simulink model "FOC_simu"  (R2018b)
settings: Solver=FixedStepDiscrete  StartTime=0.0  StopTime=inf  FixedStep=4e-6  RelTol=1e-3
undefined symbols (not defined in the file or in its folder): sigbuilder_block
libraries: simulink x7, powerlib x4
settings Model: Creator=Administrator  LastModifiedBy=nie.fei
settings DataIOCC: LimitDataPoints=on
settings OptimizationCC: BlockReduction=off  DefaultParameterBehavior=Inlined  DefaultUnderspecifiedDataType=single  LifeSpan=1
settings DebuggingCC: SignalInfNanChecking=warning  UnderspecifiedInitializationDetection=Classic  MergeDetectMultiDrivingBlocksExec=none  MultiTaskCondExecSysMsg=warning  MultiTaskRateTransMsg=warning  ParameterPrecisionLossMsg=none  SFUnexpectedBacktrackingDiag=warning  SFNoUnconditionalDefaultTransitionDiag=warning  SFExecutionAtInitializationDiag=none
settings HardwareCC: ProdBitPerPointer=32  ProdBitPerSizeT=32  ProdBitPerPtrDiffT=32  ProdLargestAtomicInteger=Long  ProdLargestAtomicFloat=Double  ProdWordSize=32  ProdHWDeviceType=ARM Compatible->ARM Cortex
settings ModelReferenceCC: PropagateSignalLabelsOutOfModel=off
settings SFSimCC: SimUseLocalCustomCode=off  MATLABDynamicMemAlloc=off
settings RTWCC: SystemTargetFile=ert.tlc  GenCodeOnly=on  PackageName=AccPedal  TemplateMakefile=ert_default_tmf  GenerateReport=on  RTWVerbose=off  RTWUseLocalCustomCode=off  IncludeHyperlinkInReport=on  LaunchReport=on
settings CodeAppCC: IgnoreCustomStorageClasses=off  MaxIdLength=63  StateflowObjectComments=on
settings ERTTargetCC: TargetLangStandard=C99 (ISO)  MultiwordLength=2048  SupportNonFinite=off  ExtModeTransport=1  ExtModeMexFile=ext_serial_win32_comm  ERTCustomFileTemplate=example_file_process.tlc  ConvertIfToSwitch=off  SuppressUnreachableDefaultCases=off
settings ConfigComp: CovMetricSettings=dw  CovHtmlReporting=on  CovSaveCumulativeToWorkspaceVar=on  CovSaveSingleToWorkspaceVar=on  CovExternalEMLEnable=off  DVMaxProcessTime=600  DVMaxTestCaseSteps=500  DVTestSuiteOptimization=CombinedObjectives (Nonlinear Extended)  DVSaveReport=on
settings SimscapeCC: SimscapeNormalizeSystem=off

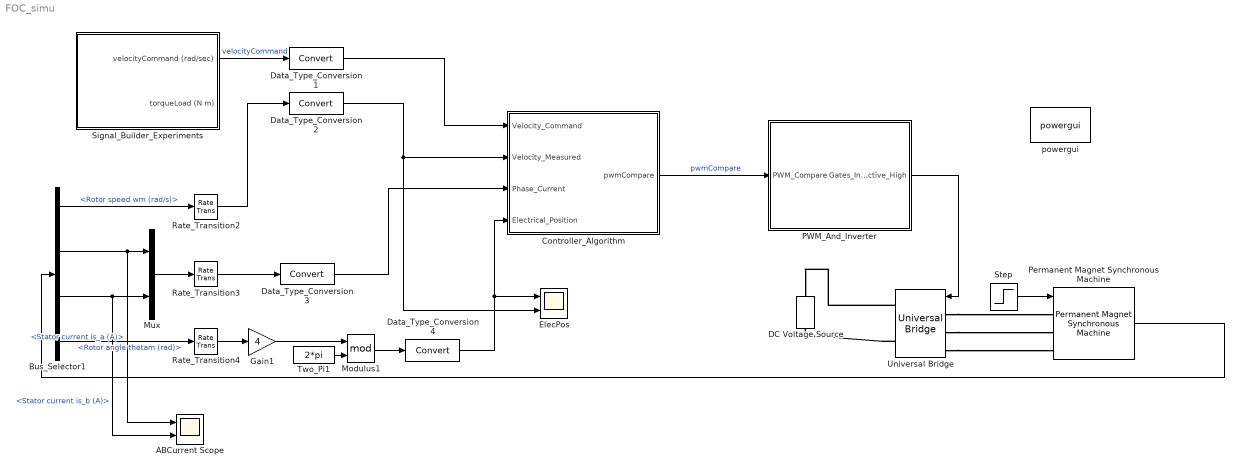
== system FOC_simu ==
  ABCurrent Scope : Scope  NumInputPorts=2
  Bus_Selector1 : BusSelector  OutputSignals=Rotor speed wm (rad/s),Stator current is_a (A),Stator current is_b (A),Rotor angle thetam (rad)
  Controller_Algorithm : Subsystem
  DC Voltage Source : powerlib/Electrical Sources/DC Voltage Source  Amplitude=24  Measurements=None
      settings: AttributesFormatString=%<Amplitude>
  Data_Type_Conversion{1..4} (4 alike) : DataTypeConversion
  ElecPos : Scope  NumInputPorts=2
  Gain1 : Gain  Gain=4
  Modulus1 : Math  Operator=mod  SaturateOnIntegerOverflow=on
  Mux : Mux  Inputs=2
  PWM_And_Inverter : Subsystem  VariantControl=variantPwm == enumPwm.behavior
      mask Display:
      | image('pwmAndInverterMask.png')
      | port_label('input',1,'En')
      | port_label('input',2,'Compare')
      | text(0.98, 0.88, 'G', 'HorizontalAlignment', 'Right')
      | text(0.98, 0.62, 'A', 'HorizontalAlignment', 'Right')
      | text(0.98, 0.38, 'B', 'HorizontalAlignment', 'Right')
      | text(0.98, 0.12, 'C', 'HorizontalAlignment', 'Right')
  Permanent Magnet Synchronous Machine : powerlib/Machines/Permanent Magnet Synchronous Machine  NbPhases=3  FluxDistribution=Sinusoidal  RotorType=Salient-pole  MechanicalLoad=Torque Tm  PresetModel=No  ShowDetailedParameters=on  MeasurementBus=off  Resistance=0.9  Inductance=8.5e-3  dqInductances=[0.0011 0.0011]  La=0.000395  MachineConstant=Flux linkage established by magnets (V.s)  Flux=0.0057  VoltageCst=4.1355  TorqueCst=0.0342  Flat=120  Mechanical=[2.400927680000000e-06 1.333630000000000e-05 4 0]  PolePairs=4  InitialConditions=[0,0, 0,0]  InitialConditions5ph=[0 0 0 0 0 0]  TsPowergui=0  TsBlock=-1  RefAngle=Aligned with phase A axis (original Park)
      settings: SourceProductName=Simscape Power Systems
  Rate_Transition2 : RateTransition  Integrity=off  Deterministic=off
  Rate_Transition3 : RateTransition  Integrity=off  Deterministic=off
  Rate_Transition4 : RateTransition  Integrity=off  Deterministic=off
  Signal_Builder_Experiments : Subsystem  Tag=STV Subsys  LoadFcn=sigbuilder_block('load');  StartFcn=sigbuilder_block('start');  StopFcn=sigbuilder_block('stop');  ClipboardFcn=sigbuilder_block('clipboard');  mask(Sigbuilder block){tuvar=[0:10]}
      mask init:
      | if ~strcmp(get_param(bdroot(gcb),'SimulationStatus'),'stopped'),tuvar = sigbuilder_block('maskInit'); end
      settings: CopyFcn=sigbuilder_block('copy');  DeleteFcn=sigbuilder_block('delete');  ModelCloseFcn=sigbuilder_block('modelClose');  PreSaveFcn=sigbuilder_block('preSave');  PauseFcn=sigbuilder_block('pause');  ContinueFcn=sigbuilder_block('continue');  NameChangeFcn=sigbuilder_block('namechange');  OpenFcn=sigbuilder_block('open',[0 30 1024.5 487.5 ]);  CloseFcn=sigbuilder_block('close');
      mask Display: plot(0, 0, 100, 100,[2, 2, 32, 32, 2], [68, 8, 8, 68, 68],[32, 2], [38, 38], [32, 19, 2],[53, 60, 44], [32, 17, 17, 2],[16, 16, 31, 31]);txt = getActiveGroup(gcbh);text(2, 100, txt,'verticalAlignment', 'top');
  Step : Step  Time=0.01  After=0
  Two_Pi1 : Constant  Value=2*pi  OutDataTypeStr=Inherit: Inherit via back propagation
  Universal Bridge : powerlib/Power Electronics/Universal Bridge  Arms=3  SnubberResistance=1e5  SnubberCapacitance=inf  Device=IGBT / Diodes  Ron=1e-3  Lon=0  ForwardVoltages="[  0  0  ]"  ForwardVoltage=0  GTOparameters=[ 10e-6 , 20e-6 ]  IGBTparameters=[ 1e-6 , 2e-6 ]  Measurements=None  Measurements_2=None  converterType=Rectifier
  powergui : powerlib/powergui  Priority=1  SimulationMode=Discrete  SampleTime=4.0e-6  frequency=60  Iterations=50  frequencyindice=0  Pbase=100e6  ErrMax=1e-4  UnitsV=kV  UnitsW=MW  buscounter=0  FunctionMessages=off  echomessages=off  EnableUseOfTLC=off  CurrentSourceSwitches=off  DisableSnubberDevices=off  DisableRonSwitches=off  DisableVfSwitches=off  DisplayEquations=off  SolverType=Tustin/Backward Euler (TBE)  Interpol=off  ExternalGateDelay=off  methode=off  Ts=0  x0status=blocks  SPID=off  SwTol=0  HookPort=off  RestoreLinks=warning  ResistiveCurrentMeasurement=off  Frange=[0:2:500]  Ylog=off  Xlog=on  ShowGrid=off  save=off  variable=ZData  structure=0  ZoomFFT=on  StartTime=0.0  cycles=1  DisplayStyle=1  fundamental=60  FreqAxis=off  MaxFrequency=1000  frequencyindicesteady=1  RmsSteady=1  display=off
  wires:
  Step/1 -> Permanent Magnet Synchronous Machine/1
  Permanent Magnet Synchronous Machine/1 -> Bus_Selector1/1
  Rate_Transition4/1 -> Gain1/1
  Bus_Selector1/2 -> Mux/1, ABCurrent Scope/1  "<Stator current is_a (A)>"
  Mux/1 -> Rate_Transition3/1
  Bus_Selector1/3 -> Mux/2, ABCurrent Scope/2  "<Stator current is_b (A)>"
  Data_Type_Conversion3/1 -> Controller_Algorithm/3(Phase_Current)
  Rate_Transition3/1 -> Data_Type_Conversion3/1
  Bus_Selector1/4 -> Rate_Transition4/1  "<Rotor angle thetam (rad)>"
  Bus_Selector1/1 -> Rate_Transition2/1  "<Rotor speed wm (rad/s)>"
  Rate_Transition2/1 -> Data_Type_Conversion2/1
  Signal_Builder_Experiments/1(velocityCommand (rad/sec)) -> Data_Type_Conversion1/1  "velocityCommand"
  Gain1/1 -> Modulus1/1
  Modulus1/1 -> Data_Type_Conversion4/1
  Controller_Algorithm/1(pwmCompare) -> PWM_And_Inverter/1(PWM_Compare)  "pwmCompare"
  PWM_And_Inverter/1(Gates_Individual_Active_High) -> Universal Bridge/1
  Data_Type_Conversion1/1 -> Controller_Algorithm/1(Velocity_Command)
  Data_Type_Conversion4/1 -> ElecPos/1, Controller_Algorithm/4(Electrical_Position)
  Two_Pi1/1 -> Modulus1/2
  Data_Type_Conversion2/1 -> ElecPos/2, Controller_Algorithm/2(Velocity_Measured)
  connections:
  Universal Bridge/LConn1 -- Permanent Magnet Synchronous Machine/LConn1
  Universal Bridge/RConn1 -- DC Voltage Source/RConn1
  Universal Bridge/RConn2 -- DC Voltage Source/LConn1
  Universal Bridge/LConn2 -- Permanent Magnet Synchronous Machine/LConn2
  Universal Bridge/LConn3 -- Permanent Magnet Synchronous Machine/LConn3

== system FOC_simu/Controller_Algorithm ==
  Velocity_Command : Inport  OutDataTypeStr=single
  Velocity_Measured : Inport  Port=2  OutDataTypeStr=single
  Phase_Current : Inport  Port=3  OutDataTypeStr=single
  Electrical_Position : Inport  Port=4  OutDataTypeStr=single
  CurrentControl : Subsystem  TreatAsAtomicUnit=on  SystemSampleTime=200e-6  RTWFcnName=CurrentControl_Co  RTWFileName=CurrentControl
      settings: RTWSystemCode=Nonreusable function  RTWFcnNameOpts=User specified  RTWFileNameOpts=User specified
      settings: AttributesFormatString=|
      | ---------------------------------------
      | SampeTime = %<SystemSampleTime>
  SpeedControl : Subsystem  TreatAsAtomicUnit=on  SystemSampleTime=0.01  RTWFcnName=SpeedControl_Co  RTWFileName=SpeedControl
      settings: RTWSystemCode=Nonreusable function  RTWFcnNameOpts=User specified  RTWFileNameOpts=User specified
      settings: AttributesFormatString=|
      | ---------------------------------------
      | SampeTime = %<SystemSampleTime>
  pwmCompare : Outport
  wires:
  Velocity_Command/1 -> SpeedControl/1(Velocity_Command)
  Velocity_Measured/1 -> SpeedControl/2(Velocity_Measured)  "speed"
  Phase_Current/1 -> CurrentControl/1(Phase_Current)
  Electrical_Position/1 -> CurrentControl/3(Electrical_Position)
  CurrentControl/1(pwmCompare) -> pwmCompare/1
  SpeedControl/1(current_Iq) -> CurrentControl/2(current_Iq)

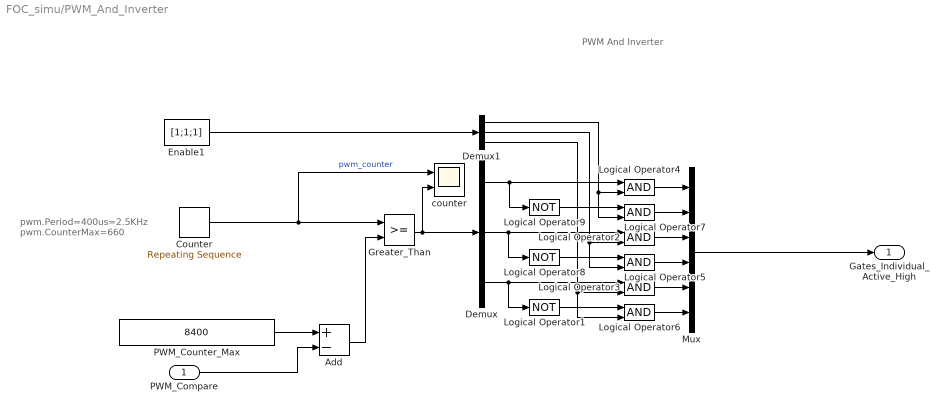
== system FOC_simu/PWM_And_Inverter ==
  note: pwm.Period=400us=2.5KHz
      | pwm.CounterMax=660
  note: PWM And Inverter
  PWM_Compare : Inport
  Add : Sum  Inputs=+-  OutDataTypeStr=Inherit: Same as first input
  Counter : simulink/Sources/Repeating Sequence  rep_seq_t=0.00005 * [0 0.5 1]  rep_seq_y=8400 * [0 1 0]
      settings: AttributesFormatString=|
      | ---------------------------------------
      | Time = %<rep_seq_t>
      | Values = %<rep_seq_y>
  Demux : Demux  Outputs=3
  Demux1 : Demux  Outputs=3
  Enable1 : Constant  Value=[1;1;1]
  Greater_Than : RelationalOperator  OutDataTypeStr=boolean  RndMeth=Nearest
  Logical Operator1 : Logic  Operator=NOT  IconShape=distinctive  AllPortsSameDT=off  OutDataTypeStr=boolean
  Logical Operator{2..7} (6 alike) : Logic  IconShape=distinctive  AllPortsSameDT=off  OutDataTypeStr=boolean
  Logical Operator8 : Logic  Operator=NOT  IconShape=distinctive  AllPortsSameDT=off  OutDataTypeStr=boolean
  Logical Operator9 : Logic  Operator=NOT  IconShape=distinctive  AllPortsSameDT=off  OutDataTypeStr=boolean
  Mux : Mux  Inputs=6
  PWM_Counter_Max : Constant  Value=8400  OutDataTypeStr=uint16
  counter : Scope  NumInputPorts=2
  Gates_Individual_Active_High : Outport
  wires:
  Mux/1 -> Gates_Individual_Active_High/1
  Counter/1 -> counter/1, Greater_Than/1  "pwm_counter"
  Demux/2 -> Logical Operator2/1, Logical Operator8/1
  Logical Operator1/1 -> Logical Operator6/1
  Logical Operator3/1 -> Mux/5
  Demux/1 -> Logical Operator9/1, Logical Operator4/1
  Logical Operator5/1 -> Mux/4
  Logical Operator6/1 -> Mux/6
  Demux1/1 -> Logical Operator4/2, Logical Operator7/2
  Demux1/3 -> Logical Operator6/2, Logical Operator3/2
  Logical Operator9/1 -> Logical Operator7/1
  Demux1/2 -> Logical Operator5/2, Logical Operator2/2
  Logical Operator8/1 -> Logical Operator5/1
  Logical Operator7/1 -> Mux/2
  Logical Operator4/1 -> Mux/1
  Demux/3 -> Logical Operator3/1, Logical Operator1/1
  Logical Operator2/1 -> Mux/3
  Enable1/1 -> Demux1/1
  Greater_Than/1 -> counter/2, Demux/1
  PWM_Compare/1 -> Add/2
  PWM_Counter_Max/1 -> Add/1
  Add/1 -> Greater_Than/2

== system FOC_simu/Signal_Builder_Experiments ==
  Demux : Demux  Tag=STV Demux  Outputs=2
  FromWs : FromWorkspace  Tag=STV FromWs  VariableName=tuvar
      SigBuilderData=|
      | dataSet(1).timeRange = [0 4.5]
      | dataSet(1).name = '150 rad/sec, no load'
      | dataSet(2).timeRange = [0 1]
      | dataSet(2).name = '+/-1 150 rad/sec, no load'
      | sbobj.Name = 'Signal Builder'
      | sbobj.Groups(1).Name = '150 rad/sec, no load'
      | sbobj.Groups(1).Signals(1).Name = 'velocityCommand (rad/sec)'
      | sbobj.Groups(1).Signals(1).XData = [0 0.05 0.5 0.7 1.1 3.7 3.9 3.9 4.3 4.3 4.5]
      | sbobj.Groups(1).Signals(1).YData = [0 0 150 200 200 200 200 100 100 150 150]
      | sbobj.Groups(1).Signals(2).Name = 'torqueLoad (N m)'
      | sbobj.Groups(1).Signals(2).XData = [0 4.5]
      | sbobj.Groups(1).Signals(2).YData = [0 0]
      | sbobj.Groups(1).TimeRange = [0 4.5]
      | sbobj.Groups(2).Name = '+/-1 150 rad/sec, no load'
      | sbobj.Groups(2).Signals(1).Name = 'velocityCommand (rad/sec)'
      | sbobj.Groups(2).Signals(1).XData = [0 0.05 0.05 0.5 0.5 0.8 0.8 1]
      | sbobj.Groups(2).Signals(1).YData = [0 0 150 150 -150 -150 0 0]
      | sbobj.Groups(2).Signals(2).Name = 'torqueLoad (N m)'
      | sbobj.Groups(2).Signals(2).XData = [0 1]
      | sbobj.Groups(2).Signals(2).YData = [0 0]
      | sbobj.Groups(2).TimeRange = [0 1]
  velocityCommand (rad/sec) : Outport  Tag=STV Outport
  torqueLoad (N m) : Outport  Tag=STV Outport  Port=2
  wires:
  Demux/2 -> torqueLoad (N m)/1
  Demux/1 -> velocityCommand (rad/sec)/1
  FromWs/1 -> Demux/1

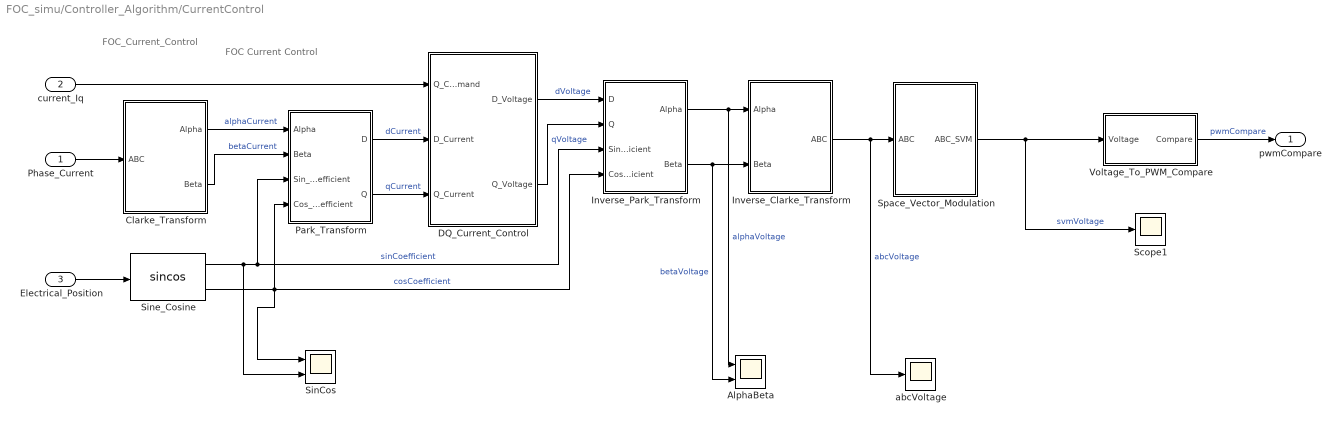
== system FOC_simu/Controller_Algorithm/CurrentControl ==
  note: FOC Current Control
  note: FOC_Current_Control
  Phase_Current : Inport  OutDataTypeStr=single
  current_Iq : Inport  Port=2
  Electrical_Position : Inport  Port=3  OutDataTypeStr=single
  AlphaBeta : Scope  NumInputPorts=2
  Clarke_Transform : Subsystem
      mask Display:
      | port_label('input',1,'ABC')
      | port_label('output',1,'\alpha','texmode', 'on')
      | port_label('output',2,'\beta','texmode', 'on')
  DQ_Current_Control : Subsystem
  Inverse_Clarke_Transform : Subsystem  VariantControl=INVERSE_CLARKE_TRANSFORM
      mask Display:
      | port_label('input',1,'\alpha','texmode', 'on')
      | port_label('input',2,'\beta','texmode', 'on')
      | port_label('output',1,'ABC')
  Inverse_Park_Transform : Subsystem
      mask Display:
      | port_label('input',1,'D')
      | port_label('input',2,'Q')
      | port_label('input',3,'Sin')
      | port_label('input',4,'Cos')
      | port_label('output',1,'\alpha','texmode', 'on')
      | port_label('output',2,'\beta','texmode', 'on')
  Park_Transform : Subsystem
      mask Display:
      | port_label('input',1,'\alpha','texmode', 'on')
      | port_label('input',2,'\beta','texmode', 'on')
      | port_label('input',3,'Sin')
      | port_label('input',4,'Cos')
      | port_label('output',1,'D')
      | port_label('output',2,'Q')
  Scope1 : Scope
  SinCos : Scope  NumInputPorts=2
  Sine_Cosine : Trigonometry  Operator=sincos
  Space_Vector_Modulation : Subsystem  VariantControl=SpaceVectorModulation_JB
      mask Display:
      | plot([0.000 0.020 0.041 0.061 0.082 0.102 0.122 0.143 0.163 0.184 0.204 0.224 0.245 0.265 0.286 0.306 0.327 0.347 0.367 0.388 0.408 0.429 0.449 0.469 0.490 0.510 0.531 0.551 0.571 0.592 0.612 0.633 0.653 0.673 0.694 0.714 0.735 0.755 0.776 0.796 0.816 0.837 0.857 0.878 0.898 0.918 0.939 0.959 0.980 1.000 ], ...
      |      [0.500 0.586 0.671 0.753 0.831 0.858 0.875 0.885 0.890 0.887 0.879 0.864 0.844 0.855 0.872 0.884 0.889 0.888 0.881 0.867 0.847 0.793 0.713 0.629 0.543 0.457 0.371 0.287 0.207 0.153 0.133 0.119 0.112 0.111 0.116 0.128 0.145 0.156 0.136 0.121 0.113 0.110 0.115 0.125 0.142 0.169 0.247 0.329 0.414 0.500 ])
  Voltage_To_PWM_Compare : Subsystem
  abcVoltage : Scope
  pwmCompare : Outport
  wires:
  Clarke_Transform/2(Beta) -> Park_Transform/2(Beta)  "betaCurrent"
  Inverse_Clarke_Transform/1(ABC) -> abcVoltage/1, Space_Vector_Modulation/1(ABC)  "abcVoltage"
  Phase_Current/1 -> Clarke_Transform/1(ABC)
  Electrical_Position/1 -> Sine_Cosine/1
  Inverse_Park_Transform/2(Beta) -> AlphaBeta/2, Inverse_Clarke_Transform/2(Beta)  "betaVoltage"
  Sine_Cosine/1 -> Park_Transform/3(Sin_Coefficient), Inverse_Park_Transform/3(Sin_Coefficient), SinCos/2  "sinCoefficient"
  Space_Vector_Modulation/1(ABC_SVM) -> Voltage_To_PWM_Compare/1(Voltage), Scope1/1  "svmVoltage"
  Park_Transform/1(D) -> DQ_Current_Control/2(D_Current)  "dCurrent"
  Sine_Cosine/2 -> SinCos/1, Park_Transform/4(Cos_Coefficient), Inverse_Park_Transform/4(Cos_Coefficient)  "cosCoefficient"
  Inverse_Park_Transform/1(Alpha) -> AlphaBeta/1, Inverse_Clarke_Transform/1(Alpha)  "alphaVoltage"
  Clarke_Transform/1(Alpha) -> Park_Transform/1(Alpha)  "alphaCurrent"
  Park_Transform/2(Q) -> DQ_Current_Control/3(Q_Current)  "qCurrent"
  Voltage_To_PWM_Compare/1(Compare) -> pwmCompare/1  "pwmCompare"
  DQ_Current_Control/1(D_Voltage) -> Inverse_Park_Transform/1(D)  "dVoltage"
  DQ_Current_Control/2(Q_Voltage) -> Inverse_Park_Transform/2(Q)  "qVoltage"
  current_Iq/1 -> DQ_Current_Control/1(Q_Command)

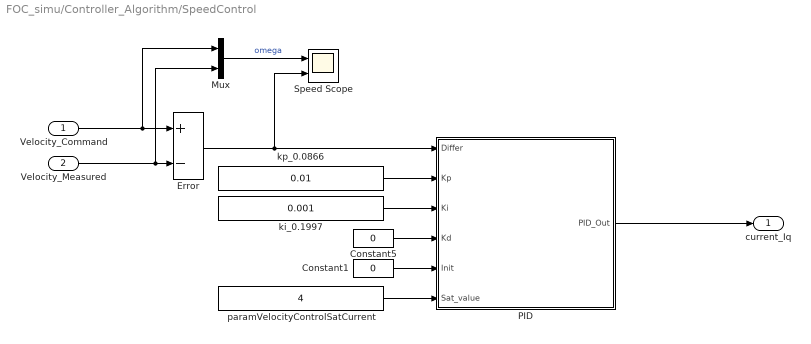
== system FOC_simu/Controller_Algorithm/SpeedControl ==
  Velocity_Command : Inport  OutDataTypeStr=single
  Velocity_Measured : Inport  Port=2  OutDataTypeStr=single
  Constant1 : Constant  Value=0  OutDataTypeStr=boolean  SampleTime=-1
  Constant5 : Constant  Value=0  OutDataTypeStr=Inherit: Inherit via back propagation  SampleTime=-1
  Error : Sum  Inputs=+-
  Mux : Mux  Inputs=2
  PID : Subsystem
  Speed Scope : Scope  NumInputPorts=2
  ki_0.1997 : Constant  Value=0.001  OutDataTypeStr=Inherit: Inherit via back propagation  SampleTime=-1
  kp_0.0866 : Constant  Value=0.01  OutDataTypeStr=Inherit: Inherit via back propagation  SampleTime=-1
  paramVelocityControlSatCurrent : Constant  Value=4  OutDataTypeStr=Inherit: Inherit via back propagation  SampleTime=-1
  current_Iq : Outport
  wires:
  PID/1(PID_Out) -> current_Iq/1
  ki_0.1997/1 -> PID/3(Ki)
  kp_0.0866/1 -> PID/2(Kp)
  Velocity_Measured/1 -> Mux/2, Error/2
  Error/1 -> Speed Scope/2, PID/1(Differ)
  Constant5/1 -> PID/4(Kd)
  Constant1/1 -> PID/5(Init)
  paramVelocityControlSatCurrent/1 -> PID/6(Sat_value)
  Mux/1 -> Speed Scope/1  "omega"
  Velocity_Command/1 -> Mux/1, Error/1

== system FOC_simu/Controller_Algorithm/CurrentControl/Clarke_Transform ==
  note: Clarke Transform
  note: Converts balanced three-phase quantities into balanced two-phase quantities.
      | The A and B phases are converted to the direct axis (alpha) component and the quadrature axis (beta) component.
      | The alpha and beta components are still dependent on time and speed.
  ABC : Inport
  A : Selector  IndexMode=Zero-based  InputPortWidth=2  IndexOptions=Index vector (dialog)  Indices=0  OutputSizes=1
  Add : Sum  OutDataTypeStr=Inherit: Same as first input
  Alpha_Gain : Gain  Gain=1/sqrt(3)
  B : Selector  IndexMode=Zero-based  InputPortWidth=2  IndexOptions=Index vector (dialog)  Indices=1  OutputSizes=1
  Beta_Gain : Gain  Gain=2/sqrt(3)
  Alpha : Outport
  Beta : Outport  Port=2
  wires:
  Add/1 -> Beta/1
  B/1 -> Beta_Gain/1
  Beta_Gain/1 -> Add/2
  ABC/1 -> A/1, B/1
  Alpha_Gain/1 -> Add/1
  A/1 -> Alpha_Gain/1, Alpha/1

== system FOC_simu/Controller_Algorithm/CurrentControl/DQ_Current_Control ==
  note: DQ Current Control
  Q_Command : Inport
  D_Current : Inport  Port=2
  Q_Current : Inport  Port=3
  Constant1 : Constant  Value=0.09  OutDataTypeStr=Inherit: Inherit via back propagation  SampleTime=-1
  Constant5 : Constant  Value=1.2  OutDataTypeStr=Inherit: Inherit via back propagation  SampleTime=-1
  D_Command : Constant  Value=0  OutDataTypeStr=single  SampleTime=-1
  D_Current_Control : Subsystem
  Q_Current_Control : Subsystem
  D_Voltage : Outport
  Q_Voltage : Outport  Port=2
  wires:
  Q_Current_Control/1(Voltage_Vq) -> Q_Voltage/1  "VQ"
  D_Current_Control/1(Voltage_Vd) -> D_Voltage/1  "VD"
  D_Command/1 -> D_Current_Control/1(Current_Command)  "IDcmd"
  Q_Command/1 -> Q_Current_Control/1(Current_Command)  "IQcmd"
  Q_Current/1 -> Q_Current_Control/2(Current_Measured)  "IQmea"
  D_Current/1 -> D_Current_Control/2(Current_Measured)  "IDmea"
  Constant5/1 -> Q_Current_Control/3(Current_Kp), D_Current_Control/3(Current_Kp)
  Constant1/1 -> Q_Current_Control/4(Current_Ki), D_Current_Control/4(Current_Ki)

== system FOC_simu/Controller_Algorithm/CurrentControl/Inverse_Clarke_Transform ==
  note: Inverse Clarke Transform
  note: Converts direct axis (alpha) component and the quadrature axis (beta) component to balanced three-phase quantities
      | The alpha and beta components are dependent on time and speed.
  Alpha : Inport
  Beta : Inport  Port=2
  Add : Sum  Inputs=-+  OutDataTypeStr=Inherit: Same as first input
  Add1 : Sum  Inputs=--  OutDataTypeStr=Inherit: Same as first input
  Gain : Gain  Gain=1/2
  Gain1 : Gain  Gain=sqrt(3)/2
  Mux : Mux  Inputs=3
  ABC : Outport
  wires:
  Gain/1 -> Add1/1, Add/1
  Gain1/1 -> Add1/2, Add/2
  Add/1 -> Mux/2
  Add1/1 -> Mux/3
  Beta/1 -> Gain1/1
  Alpha/1 -> Mux/1, Gain/1
  Mux/1 -> ABC/1

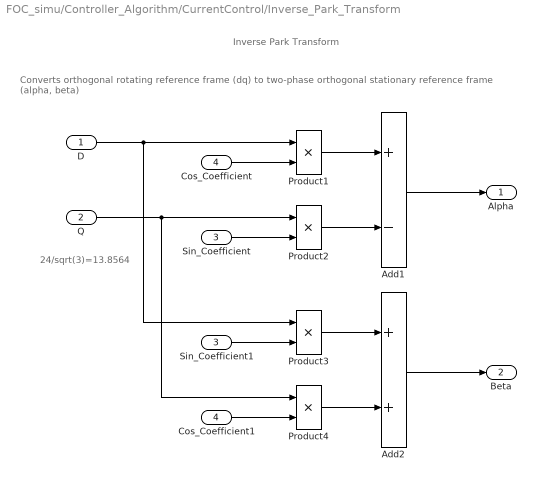
== system FOC_simu/Controller_Algorithm/CurrentControl/Inverse_Park_Transform ==
  note: Inverse Park Transform
  note: Converts orthogonal rotating reference frame (dq) to two-phase orthogonal stationary reference frame (alpha, beta)
  note: 24/sqrt(3)=13.8564
  D : Inport
  Q : Inport  Port=2
  Sin_Coefficient : Inport  Port=3
  Cos_Coefficient : Inport  Port=4
  Add1 : Sum  Inputs=+-  OutDataTypeStr=Inherit: Same as first input
  Add2 : Sum  OutDataTypeStr=Inherit: Same as first input
  Cos_Coefficient1 : InportShadow  Port=4
  Product{1..4} (4 alike) : Product  RndMeth=Simplest
  Sin_Coefficient1 : InportShadow  Port=3
  Alpha : Outport
  Beta : Outport  Port=2
  wires:
  Add2/1 -> Beta/1
  Add1/1 -> Alpha/1
  Product3/1 -> Add2/1
  Product4/1 -> Add2/2
  Product1/1 -> Add1/1
  Product2/1 -> Add1/2
  Cos_Coefficient1/1 -> Product4/2
  Sin_Coefficient/1 -> Product2/2
  D/1 -> Product3/1, Product1/1
  Q/1 -> Product2/1, Product4/1
  Sin_Coefficient1/1 -> Product3/2
  Cos_Coefficient/1 -> Product1/2

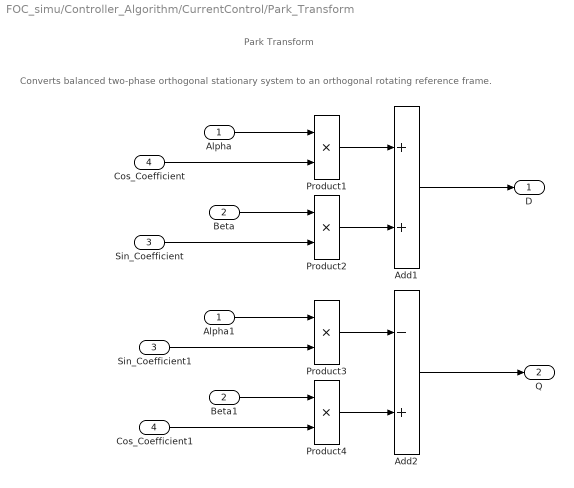
== system FOC_simu/Controller_Algorithm/CurrentControl/Park_Transform ==
  note: Park Transform
  note: Converts balanced two-phase orthogonal stationary system to an orthogonal rotating reference frame.
  Alpha : Inport
  Beta : Inport  Port=2
  Sin_Coefficient : Inport  Port=3
  Cos_Coefficient : Inport  Port=4
  Add1 : Sum  OutDataTypeStr=Inherit: Same as first input
  Add2 : Sum  Inputs=-+  OutDataTypeStr=Inherit: Same as first input
  Alpha1 : InportShadow
  Beta1 : InportShadow  Port=2
  Cos_Coefficient1 : InportShadow  Port=4
  Product{1..4} (4 alike) : Product  RndMeth=Simplest
  Sin_Coefficient1 : InportShadow  Port=3
  D : Outport
  Q : Outport  Port=2
  wires:
  Product3/1 -> Add2/1
  Product4/1 -> Add2/2
  Product1/1 -> Add1/1
  Product2/1 -> Add1/2
  Alpha1/1 -> Product3/1
  Sin_Coefficient1/1 -> Product3/2
  Cos_Coefficient1/1 -> Product4/2
  Beta1/1 -> Product4/1
  Alpha/1 -> Product1/1
  Cos_Coefficient/1 -> Product1/2
  Beta/1 -> Product2/1
  Sin_Coefficient/1 -> Product2/2
  Add1/1 -> D/1
  Add2/1 -> Q/1

== system FOC_simu/Controller_Algorithm/CurrentControl/Space_Vector_Modulation ==
  note: Space Vector Modulation
  ABC : Inport
  Add : Sum
  Add1 : Sum  Inputs=+-
  Gain : Gain  Gain=0.5  OutDataTypeStr=Inherit: Same as input
  Max : MinMax  Function=max
  Min : MinMax
  ABC_SVM : Outport
  wires:
  Add/1 -> Gain/1
  Max/1 -> Add/1
  Min/1 -> Add/2
  Gain/1 -> Add1/2
  ABC/1 -> Min/1, Max/1, Add1/1
  Add1/1 -> ABC_SVM/1

== system FOC_simu/Controller_Algorithm/CurrentControl/Voltage_To_PWM_Compare ==
  note: paramPwmCompareMax=660
  note: -12~+12
  note: ==>paramPwmComparePerVolt=27.5==>-330~+330
  note: 330
  note: 0~660
  note: Voltage To PWM Compare
  note: ==>paramPwmComparePerVolt=350==>-4200~+4200
  Voltage : Inport
  Add : Sum  OutDataTypeStr=Inherit: Inherit via back propagation
  Data_Type_Conversion : DataTypeConversion  OutDataTypeStr=uint16  LockScale=on
  Saturation : Saturate  UpperLimit=8400  LowerLimit=0
      settings: AttributesFormatString=|
      | --------------------------------
      | Upper Limit = %<UpperLimit>
      | Lower Limit = %<LowerLimit>
  Slope : Gain  Gain=350
      settings: AttributesFormatString=|
      | ----------------------------------------
      | Gain = %<Gain>
  paramPwmCompareAtZeroVolt : Constant  Value=4200  OutDataTypeStr=Inherit: Inherit via back propagation  SampleTime=-1
  Compare : Outport
  wires:
  Data_Type_Conversion/1 -> Compare/1  "pwmCompare"
  Voltage/1 -> Slope/1  "phaseVoltage"
  Slope/1 -> Add/1
  Saturation/1 -> Data_Type_Conversion/1
  paramPwmCompareAtZeroVolt/1 -> Add/2
  Add/1 -> Saturation/1

== system FOC_simu/Controller_Algorithm/SpeedControl/PID ==
  Differ : Inport  OutDataTypeStr=single
  Kp : Inport  Port=2  OutDataTypeStr=single
  Ki : Inport  Port=3  OutDataTypeStr=single
  Kd : Inport  Port=4  OutDataTypeStr=single
  Init : Inport  Port=5  OutDataTypeStr=boolean
  Sat_value : Inport  Port=6  OutDataTypeStr=single
  Delay6 : Delay  DelayLength=1
  Regul : Subsystem
  Saturation : Subsystem
  Unary Minus2 : UnaryMinus
  PID_Out : Outport
  wires:
  Init/1 -> Regul/5(Init)
  Differ/1 -> Regul/1(Differ)
  Sat_value/1 -> Unary Minus2/1, Saturation/1(Max)
  Saturation/2(Enable_Sat) -> Delay6/1
  Saturation/1(Output) -> PID_Out/1
  Delay6/1 -> Regul/6(Enable_sat)
  Unary Minus2/1 -> Saturation/2(Min)
  Regul/2(PI_Out) -> Saturation/4(Input)
  Kd/1 -> Regul/4(Kd)
  Regul/1(Err_Out) -> Saturation/3(Err_in)
  Kp/1 -> Regul/2(Kp)
  Ki/1 -> Regul/3(Ki)

== system FOC_simu/Controller_Algorithm/CurrentControl/DQ_Current_Control/D_Current_Control ==
  note: D Current Control
  note: 24/sqrt(3)=13.8564
  Current_Command : Inport
  Current_Measured : Inport  Port=2
  Current_Kp : Inport  Port=3
  Current_Ki : Inport  Port=4
  Constant1 : Constant  Value=0  OutDataTypeStr=boolean  SampleTime=-1
  Constant5 : Constant  Value=0  OutDataTypeStr=Inherit: Inherit via back propagation  SampleTime=-1
  D current Scope : Scope  NumInputPorts=2
  Error : Sum  Inputs=+-
  PID : Subsystem  TreatAsAtomicUnit=on
  paramCurrentControlSatVoltage : Constant  Value=13.8564  OutDataTypeStr=Inherit: Inherit via back propagation  SampleTime=-1
  Voltage_Vd : Outport
  wires:
  Error/1 -> PID/1(Differ)  "currentControlError"
  Current_Command/1 -> D current Scope/1, Error/1
  Current_Measured/1 -> D current Scope/2, Error/2  "current"
  Current_Kp/1 -> PID/2(Kp)
  Constant1/1 -> PID/5(Init)
  Current_Ki/1 -> PID/3(Ki)
  Constant5/1 -> PID/4(Kd)
  paramCurrentControlSatVoltage/1 -> PID/6(Sat_value)
  PID/1(PID_Out) -> Voltage_Vd/1

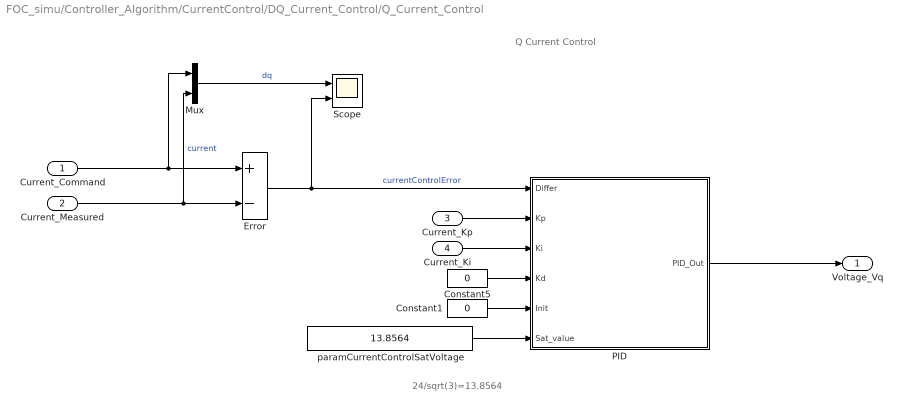
== system FOC_simu/Controller_Algorithm/CurrentControl/DQ_Current_Control/Q_Current_Control ==
  note: 24/sqrt(3)=13.8564
  note: Q Current Control
  Current_Command : Inport
  Current_Measured : Inport  Port=2
  Current_Kp : Inport  Port=3
  Current_Ki : Inport  Port=4
  Constant1 : Constant  Value=0  OutDataTypeStr=boolean  SampleTime=-1
  Constant5 : Constant  Value=0  OutDataTypeStr=Inherit: Inherit via back propagation  SampleTime=-1
  Error : Sum  Inputs=+-
  Mux : Mux  Inputs=2
  PID : Subsystem
  Scope : Scope  NumInputPorts=2
  paramCurrentControlSatVoltage : Constant  Value=13.8564  OutDataTypeStr=Inherit: Inherit via back propagation  SampleTime=-1
  Voltage_Vq : Outport
  wires:
  Current_Command/1 -> Mux/1, Error/1
  Current_Measured/1 -> Mux/2, Error/2  "current"
  Error/1 -> Scope/2, PID/1(Differ)  "currentControlError"
  Constant1/1 -> PID/5(Init)
  Current_Ki/1 -> PID/3(Ki)
  Constant5/1 -> PID/4(Kd)
  paramCurrentControlSatVoltage/1 -> PID/6(Sat_value)
  Current_Kp/1 -> PID/2(Kp)
  PID/1(PID_Out) -> Voltage_Vq/1
  Mux/1 -> Scope/1  "dq"

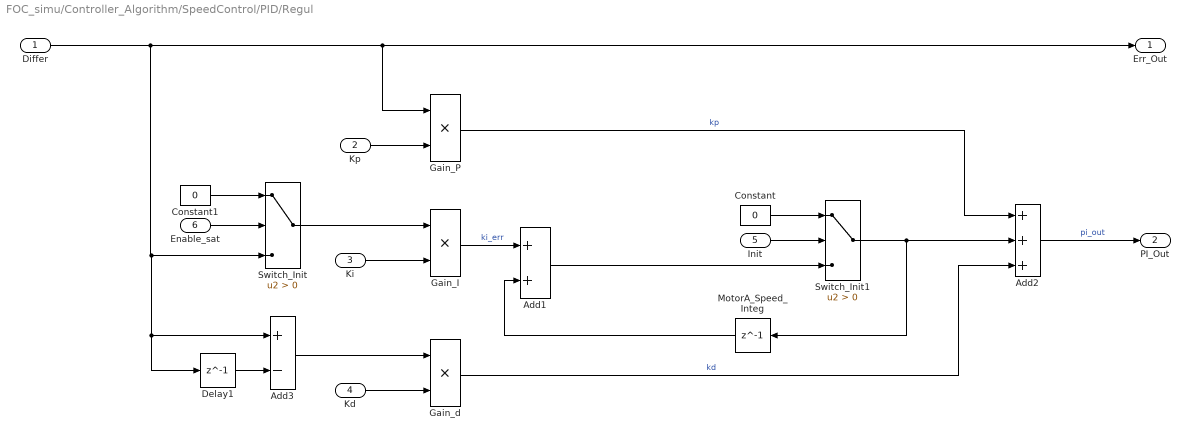
== system FOC_simu/Controller_Algorithm/SpeedControl/PID/Regul ==
  Differ : Inport
  Kp : Inport  Port=2
  Ki : Inport  Port=3
  Kd : Inport  Port=4
  Init : Inport  Port=5
  Enable_sat : Inport  Port=6
  Add1 : Sum  SaturateOnIntegerOverflow=on  InputSameDT=on  OutDataTypeStr=Inherit: Same as first input
  Add2 : Sum  Inputs=+++  OutDataTypeStr=Inherit: Inherit via back propagation  SaturateOnIntegerOverflow=on  InputSameDT=on
  Add3 : Sum  Inputs=+-  SaturateOnIntegerOverflow=on  InputSameDT=on
  Constant : Constant  Value=0  OutDataTypeStr=Inherit: Inherit via back propagation  SampleTime=-1
  Constant1 : Constant  Value=0  OutDataTypeStr=Inherit: Inherit via back propagation  SampleTime=-1
  Delay1 : Delay  DelayLength=1  InitialCondition=0
  Gain_I : Product  SaturateOnIntegerOverflow=on  RndMeth=Zero  OutDataTypeStr=Inherit: Same as first input
  Gain_P : Product  SaturateOnIntegerOverflow=on  RndMeth=Zero  OutDataTypeStr=Inherit: Same as first input
  Gain_d : Product  SaturateOnIntegerOverflow=on  RndMeth=Zero  OutDataTypeStr=Inherit: Same as first input
  MotorA_Speed_Integ : Delay  DelayLength=1  InitialCondition=0
  Switch_Init : Switch  Criteria=u2 > Threshold
  Switch_Init1 : Switch  Criteria=u2 > Threshold  OutDataTypeStr=Inherit: Inherit via back propagation  InputSameDT=on
  Err_Out : Outport  InitialOutput=0
  PI_Out : Outport  Port=2  InitialOutput=0
  wires:
  Kd/1 -> Gain_d/2
  Gain_d/1 -> Add2/3  "kd"
  Add3/1 -> Gain_d/1
  Delay1/1 -> Add3/2
  Constant/1 -> Switch_Init1/1
  Add1/1 -> Switch_Init1/3
  Enable_sat/1 -> Switch_Init/2
  Constant1/1 -> Switch_Init/1
  Init/1 -> Switch_Init1/2
  Gain_I/1 -> Add1/1  "ki_err"
  Gain_P/1 -> Add2/1  "kp"
  Differ/1 -> Err_Out/1, Gain_P/1, Switch_Init/3, Add3/1, Delay1/1
  Add2/1 -> PI_Out/1  "pi_out"
  Switch_Init1/1 -> MotorA_Speed_Integ/1, Add2/2
  MotorA_Speed_Integ/1 -> Add1/2
  Kp/1 -> Gain_P/2
  Ki/1 -> Gain_I/2
  Switch_Init/1 -> Gain_I/1

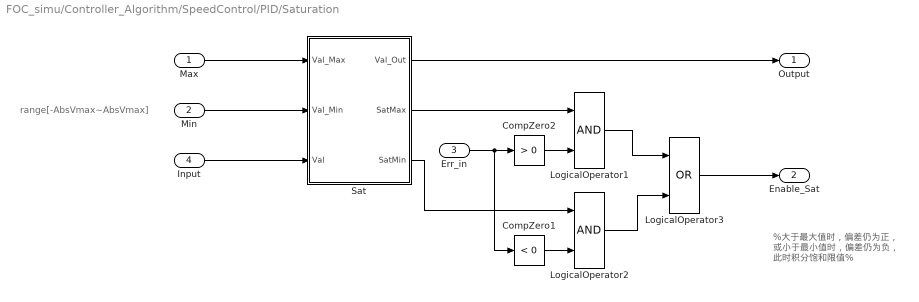
== system FOC_simu/Controller_Algorithm/SpeedControl/PID/Saturation ==
  note: %大于最大值时，偏差仍为正，
      | 或小于最小值时，偏差仍为负，
      | 此时积分饱和限值%
  note: range[-AbsVmax~AbsVmax]
  Max : Inport
  Min : Inport  Port=2
  Err_in : Inport  Port=3
  Input : Inport  Port=4
  CompZero1 : simulink/Logic and Bit Operations/Compare To Zero  relop=<  OutDataTypeStr=boolean
  CompZero2 : simulink/Logic and Bit Operations/Compare To Zero  relop=>  OutDataTypeStr=boolean
  LogicalOperator1 : Logic  OutDataTypeStr=boolean
  LogicalOperator2 : Logic  OutDataTypeStr=boolean
  LogicalOperator3 : Logic  Operator=OR  OutDataTypeStr=boolean
  Sat : Subsystem
  Output : Outport  InitialOutput=0
  Enable_Sat : Outport  Port=2  InitialOutput=0
  wires:
  Max/1 -> Sat/1(Val_Max)
  Input/1 -> Sat/3(Val)
  Min/1 -> Sat/2(Val_Min)
  Sat/1(Val_Out) -> Output/1
  Sat/2(SatMax) -> LogicalOperator1/1
  Sat/3(SatMin) -> LogicalOperator2/1
  Err_in/1 -> CompZero1/1, CompZero2/1
  CompZero2/1 -> LogicalOperator1/2
  CompZero1/1 -> LogicalOperator2/2
  LogicalOperator1/1 -> LogicalOperator3/1
  LogicalOperator2/1 -> LogicalOperator3/2
  LogicalOperator3/1 -> Enable_Sat/1

== system FOC_simu/Controller_Algorithm/CurrentControl/DQ_Current_Control/D_Current_Control/PID ==
  Differ : Inport  OutDataTypeStr=single
  Kp : Inport  Port=2  OutDataTypeStr=single
  Ki : Inport  Port=3  OutDataTypeStr=single
  Kd : Inport  Port=4  OutDataTypeStr=single
  Init : Inport  Port=5  OutDataTypeStr=boolean
  Sat_value : Inport  Port=6  OutDataTypeStr=single
  Delay6 : Delay  DelayLength=1
  Regul : Subsystem
  Saturation : Subsystem
  Unary Minus2 : UnaryMinus
  PID_Out : Outport
  wires:
  Init/1 -> Regul/5(Init)
  Differ/1 -> Regul/1(Differ)
  Sat_value/1 -> Unary Minus2/1, Saturation/1(Max)
  Saturation/2(Enable_Sat) -> Delay6/1
  Saturation/1(Output) -> PID_Out/1
  Delay6/1 -> Regul/6(Enable_sat)
  Unary Minus2/1 -> Saturation/2(Min)
  Regul/2(PI_Out) -> Saturation/4(Input)
  Kd/1 -> Regul/4(Kd)
  Regul/1(Err_Out) -> Saturation/3(Err_in)
  Kp/1 -> Regul/2(Kp)
  Ki/1 -> Regul/3(Ki)

== system FOC_simu/Controller_Algorithm/CurrentControl/DQ_Current_Control/Q_Current_Control/PID ==
  Differ : Inport  OutDataTypeStr=single
  Kp : Inport  Port=2  OutDataTypeStr=single
  Ki : Inport  Port=3  OutDataTypeStr=single
  Kd : Inport  Port=4  OutDataTypeStr=single
  Init : Inport  Port=5  OutDataTypeStr=boolean
  Sat_value : Inport  Port=6  OutDataTypeStr=single
  Delay6 : Delay  DelayLength=1
  Regul : Subsystem
  Saturation : Subsystem
  Unary Minus2 : UnaryMinus
  PID_Out : Outport
  wires:
  Init/1 -> Regul/5(Init)
  Differ/1 -> Regul/1(Differ)
  Sat_value/1 -> Unary Minus2/1, Saturation/1(Max)
  Saturation/2(Enable_Sat) -> Delay6/1
  Saturation/1(Output) -> PID_Out/1
  Delay6/1 -> Regul/6(Enable_sat)
  Unary Minus2/1 -> Saturation/2(Min)
  Regul/2(PI_Out) -> Saturation/4(Input)
  Kd/1 -> Regul/4(Kd)
  Regul/1(Err_Out) -> Saturation/3(Err_in)
  Kp/1 -> Regul/2(Kp)
  Ki/1 -> Regul/3(Ki)

== system FOC_simu/Controller_Algorithm/SpeedControl/PID/Saturation/Sat ==
  Val_Max : Inport
  Val_Min : Inport  Port=2
  Val : Inport  Port=3
  LogicalOperator2 : Logic  Operator=NOT  OutDataTypeStr=boolean
  Relational Operator : RelationalOperator  OutDataTypeStr=boolean  RndMeth=Nearest  InputSameDT=on
  Relational Operator1 : RelationalOperator  Operator=<=  OutDataTypeStr=boolean  RndMeth=Nearest  InputSameDT=on
  Switch_Inf : Switch  Criteria=u2 > Threshold  InputSameDT=on
  Switch_Sup : Switch  Criteria=u2 > Threshold  InputSameDT=on
  Val_Out : Outport
  SatMax : Outport  Port=2  InitialOutput=0
  SatMin : Outport  Port=3  InitialOutput=0
  wires:
  Switch_Inf/1 -> Val_Out/1
  Switch_Sup/1 -> Relational Operator/1, Switch_Inf/1
  Val_Max/1 -> Switch_Sup/1, Relational Operator1/1
  Val/1 -> Switch_Sup/3, Relational Operator1/2
  Val_Min/1 -> Switch_Inf/3, Relational Operator/2
  Relational Operator/1 -> LogicalOperator2/1, Switch_Inf/2
  Relational Operator1/1 -> SatMax/1, Switch_Sup/2
  LogicalOperator2/1 -> SatMin/1

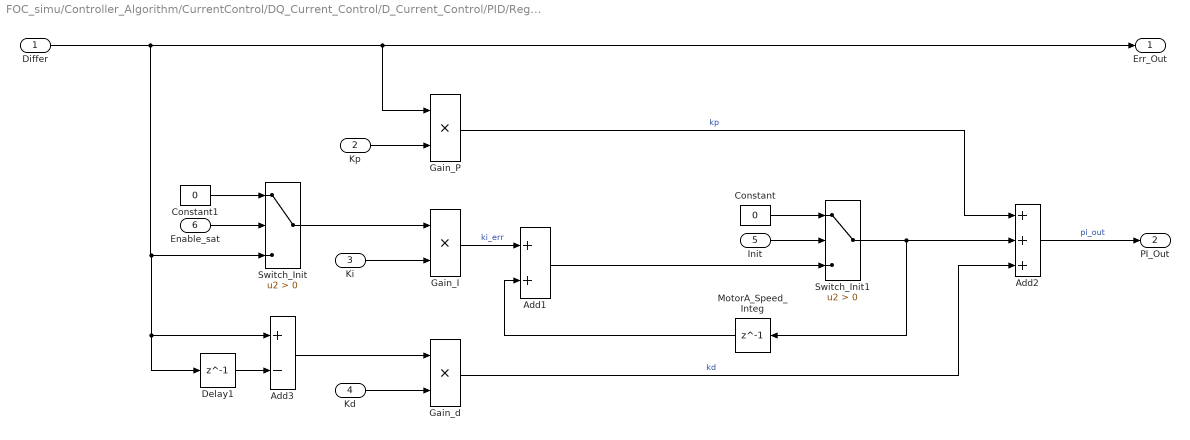
== system FOC_simu/Controller_Algorithm/CurrentControl/DQ_Current_Control/D_Current_Control/PID/Regul ==
  Differ : Inport
  Kp : Inport  Port=2
  Ki : Inport  Port=3
  Kd : Inport  Port=4
  Init : Inport  Port=5
  Enable_sat : Inport  Port=6
  Add1 : Sum  SaturateOnIntegerOverflow=on  InputSameDT=on  OutDataTypeStr=Inherit: Same as first input
  Add2 : Sum  Inputs=+++  OutDataTypeStr=Inherit: Inherit via back propagation  SaturateOnIntegerOverflow=on  InputSameDT=on
  Add3 : Sum  Inputs=+-  SaturateOnIntegerOverflow=on  InputSameDT=on
  Constant : Constant  Value=0  OutDataTypeStr=Inherit: Inherit via back propagation  SampleTime=-1
  Constant1 : Constant  Value=0  OutDataTypeStr=Inherit: Inherit via back propagation  SampleTime=-1
  Delay1 : Delay  DelayLength=1  InitialCondition=0
  Gain_I : Product  SaturateOnIntegerOverflow=on  RndMeth=Zero  OutDataTypeStr=Inherit: Same as first input
  Gain_P : Product  SaturateOnIntegerOverflow=on  RndMeth=Zero  OutDataTypeStr=Inherit: Same as first input
  Gain_d : Product  SaturateOnIntegerOverflow=on  RndMeth=Zero  OutDataTypeStr=Inherit: Same as first input
  MotorA_Speed_Integ : Delay  DelayLength=1  InitialCondition=0
  Switch_Init : Switch  Criteria=u2 > Threshold
  Switch_Init1 : Switch  Criteria=u2 > Threshold  OutDataTypeStr=Inherit: Inherit via back propagation  InputSameDT=on
  Err_Out : Outport  InitialOutput=0
  PI_Out : Outport  Port=2  InitialOutput=0
  wires:
  Kd/1 -> Gain_d/2
  Gain_d/1 -> Add2/3  "kd"
  Add3/1 -> Gain_d/1
  Delay1/1 -> Add3/2
  Constant/1 -> Switch_Init1/1
  Add1/1 -> Switch_Init1/3
  Enable_sat/1 -> Switch_Init/2
  Constant1/1 -> Switch_Init/1
  Init/1 -> Switch_Init1/2
  Gain_I/1 -> Add1/1  "ki_err"
  Gain_P/1 -> Add2/1  "kp"
  Differ/1 -> Err_Out/1, Gain_P/1, Switch_Init/3, Add3/1, Delay1/1
  Add2/1 -> PI_Out/1  "pi_out"
  Switch_Init1/1 -> MotorA_Speed_Integ/1, Add2/2
  MotorA_Speed_Integ/1 -> Add1/2
  Kp/1 -> Gain_P/2
  Ki/1 -> Gain_I/2
  Switch_Init/1 -> Gain_I/1

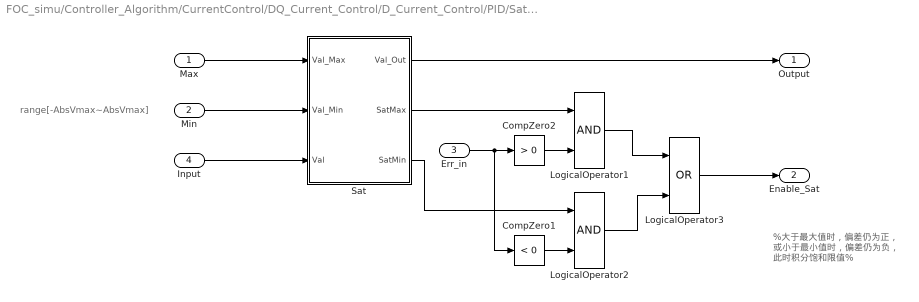
== system FOC_simu/Controller_Algorithm/CurrentControl/DQ_Current_Control/D_Current_Control/PID/Saturation ==
  note: %大于最大值时，偏差仍为正，
      | 或小于最小值时，偏差仍为负，
      | 此时积分饱和限值%
  note: range[-AbsVmax~AbsVmax]
  Max : Inport
  Min : Inport  Port=2
  Err_in : Inport  Port=3
  Input : Inport  Port=4
  CompZero1 : simulink/Logic and Bit Operations/Compare To Zero  relop=<  OutDataTypeStr=boolean
  CompZero2 : simulink/Logic and Bit Operations/Compare To Zero  relop=>  OutDataTypeStr=boolean
  LogicalOperator1 : Logic  OutDataTypeStr=boolean
  LogicalOperator2 : Logic  OutDataTypeStr=boolean
  LogicalOperator3 : Logic  Operator=OR  OutDataTypeStr=boolean
  Sat : Subsystem
  Output : Outport  InitialOutput=0
  Enable_Sat : Outport  Port=2  InitialOutput=0
  wires:
  Max/1 -> Sat/1(Val_Max)
  Input/1 -> Sat/3(Val)
  Min/1 -> Sat/2(Val_Min)
  Sat/1(Val_Out) -> Output/1
  Sat/2(SatMax) -> LogicalOperator1/1
  Sat/3(SatMin) -> LogicalOperator2/1
  Err_in/1 -> CompZero1/1, CompZero2/1
  CompZero2/1 -> LogicalOperator1/2
  CompZero1/1 -> LogicalOperator2/2
  LogicalOperator1/1 -> LogicalOperator3/1
  LogicalOperator2/1 -> LogicalOperator3/2
  LogicalOperator3/1 -> Enable_Sat/1

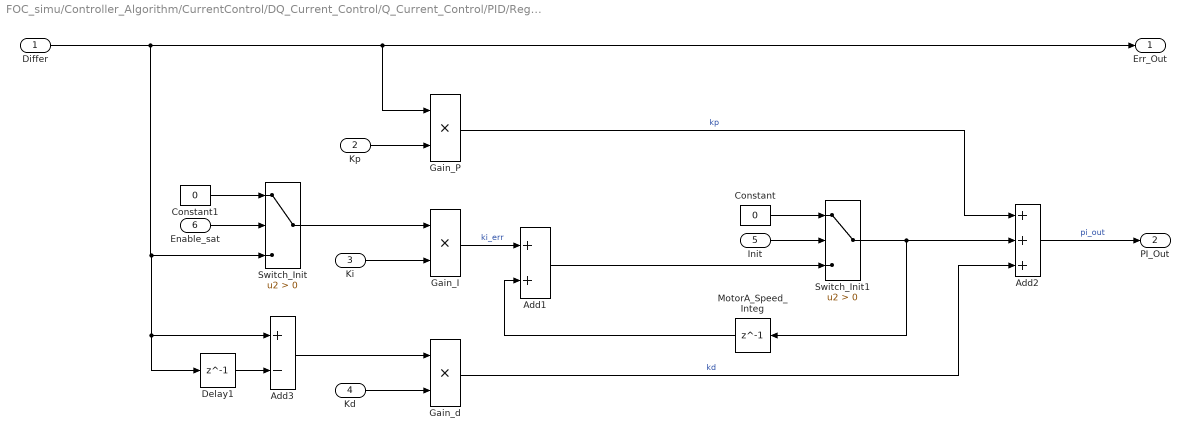
== system FOC_simu/Controller_Algorithm/CurrentControl/DQ_Current_Control/Q_Current_Control/PID/Regul ==
  Differ : Inport
  Kp : Inport  Port=2
  Ki : Inport  Port=3
  Kd : Inport  Port=4
  Init : Inport  Port=5
  Enable_sat : Inport  Port=6
  Add1 : Sum  SaturateOnIntegerOverflow=on  InputSameDT=on  OutDataTypeStr=Inherit: Same as first input
  Add2 : Sum  Inputs=+++  OutDataTypeStr=Inherit: Inherit via back propagation  SaturateOnIntegerOverflow=on  InputSameDT=on
  Add3 : Sum  Inputs=+-  SaturateOnIntegerOverflow=on  InputSameDT=on
  Constant : Constant  Value=0  OutDataTypeStr=Inherit: Inherit via back propagation  SampleTime=-1
  Constant1 : Constant  Value=0  OutDataTypeStr=Inherit: Inherit via back propagation  SampleTime=-1
  Delay1 : Delay  DelayLength=1  InitialCondition=0
  Gain_I : Product  SaturateOnIntegerOverflow=on  RndMeth=Zero  OutDataTypeStr=Inherit: Same as first input
  Gain_P : Product  SaturateOnIntegerOverflow=on  RndMeth=Zero  OutDataTypeStr=Inherit: Same as first input
  Gain_d : Product  SaturateOnIntegerOverflow=on  RndMeth=Zero  OutDataTypeStr=Inherit: Same as first input
  MotorA_Speed_Integ : Delay  DelayLength=1  InitialCondition=0
  Switch_Init : Switch  Criteria=u2 > Threshold
  Switch_Init1 : Switch  Criteria=u2 > Threshold  OutDataTypeStr=Inherit: Inherit via back propagation  InputSameDT=on
  Err_Out : Outport  InitialOutput=0
  PI_Out : Outport  Port=2  InitialOutput=0
  wires:
  Kd/1 -> Gain_d/2
  Gain_d/1 -> Add2/3  "kd"
  Add3/1 -> Gain_d/1
  Delay1/1 -> Add3/2
  Constant/1 -> Switch_Init1/1
  Add1/1 -> Switch_Init1/3
  Enable_sat/1 -> Switch_Init/2
  Constant1/1 -> Switch_Init/1
  Init/1 -> Switch_Init1/2
  Gain_I/1 -> Add1/1  "ki_err"
  Gain_P/1 -> Add2/1  "kp"
  Differ/1 -> Err_Out/1, Gain_P/1, Switch_Init/3, Add3/1, Delay1/1
  Add2/1 -> PI_Out/1  "pi_out"
  Switch_Init1/1 -> MotorA_Speed_Integ/1, Add2/2
  MotorA_Speed_Integ/1 -> Add1/2
  Kp/1 -> Gain_P/2
  Ki/1 -> Gain_I/2
  Switch_Init/1 -> Gain_I/1

== system FOC_simu/Controller_Algorithm/CurrentControl/DQ_Current_Control/Q_Current_Control/PID/Saturation ==
  note: %大于最大值时，偏差仍为正，
      | 或小于最小值时，偏差仍为负，
      | 此时积分饱和限值%
  note: range[-AbsVmax~AbsVmax]
  Max : Inport
  Min : Inport  Port=2
  Err_in : Inport  Port=3
  Input : Inport  Port=4
  CompZero1 : simulink/Logic and Bit Operations/Compare To Zero  relop=<  OutDataTypeStr=boolean
  CompZero2 : simulink/Logic and Bit Operations/Compare To Zero  relop=>  OutDataTypeStr=boolean
  LogicalOperator1 : Logic  OutDataTypeStr=boolean
  LogicalOperator2 : Logic  OutDataTypeStr=boolean
  LogicalOperator3 : Logic  Operator=OR  OutDataTypeStr=boolean
  Sat : Subsystem
  Output : Outport  InitialOutput=0
  Enable_Sat : Outport  Port=2  InitialOutput=0
  wires:
  Max/1 -> Sat/1(Val_Max)
  Input/1 -> Sat/3(Val)
  Min/1 -> Sat/2(Val_Min)
  Sat/1(Val_Out) -> Output/1
  Sat/2(SatMax) -> LogicalOperator1/1
  Sat/3(SatMin) -> LogicalOperator2/1
  Err_in/1 -> CompZero1/1, CompZero2/1
  CompZero2/1 -> LogicalOperator1/2
  CompZero1/1 -> LogicalOperator2/2
  LogicalOperator1/1 -> LogicalOperator3/1
  LogicalOperator2/1 -> LogicalOperator3/2
  LogicalOperator3/1 -> Enable_Sat/1

== system FOC_simu/Controller_Algorithm/CurrentControl/DQ_Current_Control/D_Current_Control/PID/Saturation/Sat ==
  Val_Max : Inport
  Val_Min : Inport  Port=2
  Val : Inport  Port=3
  LogicalOperator2 : Logic  Operator=NOT  OutDataTypeStr=boolean
  Relational Operator : RelationalOperator  OutDataTypeStr=boolean  RndMeth=Nearest  InputSameDT=on
  Relational Operator1 : RelationalOperator  Operator=<=  OutDataTypeStr=boolean  RndMeth=Nearest  InputSameDT=on
  Switch_Inf : Switch  Criteria=u2 > Threshold  InputSameDT=on
  Switch_Sup : Switch  Criteria=u2 > Threshold  InputSameDT=on
  Val_Out : Outport
  SatMax : Outport  Port=2  InitialOutput=0
  SatMin : Outport  Port=3  InitialOutput=0
  wires:
  Switch_Inf/1 -> Val_Out/1
  Switch_Sup/1 -> Relational Operator/1, Switch_Inf/1
  Val_Max/1 -> Switch_Sup/1, Relational Operator1/1
  Val/1 -> Switch_Sup/3, Relational Operator1/2
  Val_Min/1 -> Switch_Inf/3, Relational Operator/2
  Relational Operator/1 -> LogicalOperator2/1, Switch_Inf/2
  Relational Operator1/1 -> SatMax/1, Switch_Sup/2
  LogicalOperator2/1 -> SatMin/1

== system FOC_simu/Controller_Algorithm/CurrentControl/DQ_Current_Control/Q_Current_Control/PID/Saturation/Sat ==
  Val_Max : Inport
  Val_Min : Inport  Port=2
  Val : Inport  Port=3
  LogicalOperator2 : Logic  Operator=NOT  OutDataTypeStr=boolean
  Relational Operator : RelationalOperator  OutDataTypeStr=boolean  RndMeth=Nearest  InputSameDT=on
  Relational Operator1 : RelationalOperator  Operator=<=  OutDataTypeStr=boolean  RndMeth=Nearest  InputSameDT=on
  Switch_Inf : Switch  Criteria=u2 > Threshold  InputSameDT=on
  Switch_Sup : Switch  Criteria=u2 > Threshold  InputSameDT=on
  Val_Out : Outport
  SatMax : Outport  Port=2  InitialOutput=0
  SatMin : Outport  Port=3  InitialOutput=0
  wires:
  Switch_Inf/1 -> Val_Out/1
  Switch_Sup/1 -> Relational Operator/1, Switch_Inf/1
  Val_Max/1 -> Switch_Sup/1, Relational Operator1/1
  Val/1 -> Switch_Sup/3, Relational Operator1/2
  Val_Min/1 -> Switch_Inf/3, Relational Operator/2
  Relational Operator/1 -> LogicalOperator2/1, Switch_Inf/2
  Relational Operator1/1 -> SatMax/1, Switch_Sup/2
  LogicalOperator2/1 -> SatMin/1
